simulink model "vis_servo"  (R2020b)
settings: Solver=ode45  StartTime=0.0  StopTime=100  MaxStep=0.5e-3  RelTol=1e-11
InitFcn:
  | init
values from neighbouring files (symbols this model uses):
  C_features_0 = homtrans(inv(W_T_C_0), W_features)    [init.m]
  C_features_desired = inv(O_T_C_desired) * O_features    [init.m]
  Cdesired_T_C0 = inv(C0_T_Cdesired)    [init.m]
  lambdaT_const = 1    [init.m]
  s0 = C_features_0(:)    [init.m]
  Ts = 0.15    [init.m]    (also in test_for_c.m = 0.1)
  vMax = .5    (= 0.5)    [init.m]
  W_p_C_0 = W_T_C_0.transl'    [init.m]
  W_q_C_0 = rotm2quat(W_T_C_0.R)    [init.m]
  wMax = deg2rad(20)    [init.m]
settings Model: Creator=marco  LastModifiedBy=marco

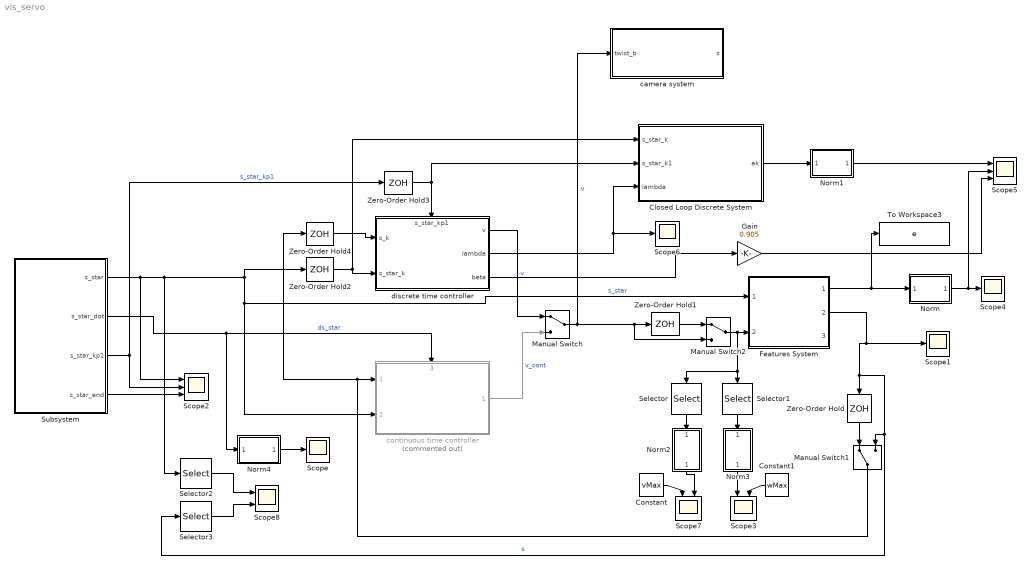
== system vis_servo ==
  Closed Loop Discrete System : Subsystem  mask{forward_action_enabled=on, Ts=Ts, e0=e0*0}
  Constant : Constant  Value=vMax
  Constant1 : Constant  Value=wMax
  Features System : Subsystem  ReferencedSubsystem=Features_System  s0=s0
  Gain : Gain  Gain=0.905
  Manual Switch : ManualSwitch
  Manual Switch1 : ManualSwitch
  Manual Switch2 : ManualSwitch
  Norm{,1..4} (5 alike) : Subsystem  ReferencedSubsystem=Norm
  Scope{,1,4,6} (4 alike) : Scope
  Scope2 : Scope  NumInputPorts=3
  Scope3 : Scope  NumInputPorts=2
  Scope5 : Scope  NumInputPorts=3
  Scope7 : Scope  NumInputPorts=2
  Scope8 : Scope  NumInputPorts=2
  Selector : Selector  InputPortWidth=6  IndexOptions=Index vector (dialog)  Indices=1:3  OutputSizes=1
  Selector1 : Selector  InputPortWidth=6  IndexOptions=Index vector (dialog)  Indices=4:6  OutputSizes=1
  Selector2 : Selector  InputPortWidth=numel(s0)  IndexOptions=Index vector (dialog)  Indices=1:3  OutputSizes=1
  Selector3 : Selector  InputPortWidth=numel(s0)  IndexOptions=Index vector (dialog)  Indices=1:3  OutputSizes=1
  Subsystem : Subsystem  mask{C_features_0=C_features_0, C_features_desired=C_features_desired, Cdesired_T_C0=Cdesired_T_C0.double, Ts=Ts, no_traj=off}
      mask prompts: C_features_0 "C_features_0 (initial features in camera frame)"; C_features_desired "C_features_desired (desired features in camera frame)"; Cdesired_T_C0 "Cdesired_T_C0 (camera initial frame w.r.t. camera desired frame)"
      mask Display:
      | disp('Ref Generator','texmode', 'on')
      | 
      | port_label('output',1,'s^*','texmode', 'on')
      | port_label('output',2,'ds^*','texmode', 'on')
      | port_label('output',3,'s^*_{k+1}','texmode', 'on')
      | port_label('output',4,'s^*_{END}','texmode', 'on')
  To Workspace3 : ToWorkspace  VariableName=e  SaveFormat=Timeseries  SampleTime=0.001
  Zero-Order Hold{,1..4} (5 alike) : ZeroOrderHold  SampleTime=Ts
  camera system : Subsystem
  continuous time controller : Subsystem  Commented=on  ReferencedSubsystem=continuous_time_controller  lambda=lambda_const  forward_action_enabled=off
      settings: PortSchema="{\"entries\":[{\"content\":{\"sides\":[{\"content\":{\"connectorIds\":[\"In1\",\"In2\"]},\"type\":\"ConnectorPlacement.EquallySpacedRectSide\",\"uuid\":\"e89226d4-baa4-4c30-af13-ff098f2ce7fc\"},{\"content\":{\"connectorIds\":[\"Out1\"],\"side\":\"RIGHT\"},\"type\":\"ConnectorPlacement.EquallySpacedRectSide\",\"uuid\":\"9d8bce32-3e74-4b83-8e79-37f4d5184f5a\"},{\"content\":{\"connectorIds\":[\"In3\"],\"side\":\"TOP\"},\"type\":\"ConnectorPlacement.EquallySpacedRectSide\",\"uuid\":\"9322580e-0316-476d-a1f3-db89d995a642\"},{\"content\":{\"connectorIds\":[],\"side\":\"HIDDEN\"},\"type\":\"ConnectorPlacement.EquallySpacedRectSide\",\"uuid\":\"a71e587c-d25e-434f-ae20-c6224730a5c7\"}]},\"type\":\"ConnectorPlacement.EquallySpacedConnector\",\"uuid\":\"c231d1ba-4204-4ba1-a9fd-ba17f6d657c2\"}],\"packageUris\":[\"http://schema.mathworks.com/mf0/Connector/R2020b\"],\"version\":\"1.0\"}"
  discrete time controller : Subsystem  mask{Ts=Ts, forward_action_enabled=on, vMax=vMax + inf, wMax=wMax + inf, use_majorant=off, use_lambda_const=on, lambdaT_const=lambdaT_const/2, use_max_analytic_lambda=off}
      settings: PortSchema="{\"entries\":[{\"content\":{\"sides\":[{\"content\":{\"connectorIds\":[\"In1\",\"In2\"]},\"type\":\"ConnectorPlacement.EquallySpacedRectSide\",\"uuid\":\"e89226d4-baa4-4c30-af13-ff098f2ce7fc\"},{\"content\":{\"connectorIds\":[\"Out1\",\"Out2\",\"Out3\"],\"side\":\"RIGHT\"},\"type\":\"ConnectorPlacement.EquallySpacedRectSide\",\"uuid\":\"9d8bce32-3e74-4b83-8e79-37f4d5184f5a\"},{\"content\":{\"connectorIds\":[\"In3\"],\"side\":\"TOP\"},\"type\":\"ConnectorPlacement.EquallySpacedRectSide\",\"uuid\":\"9322580e-0316-476d-a1f3-db89d995a642\"},{\"content\":{\"connectorIds\":[],\"side\":\"HIDDEN\"},\"type\":\"ConnectorPlacement.EquallySpacedRectSide\",\"uuid\":\"a71e587c-d25e-434f-ae20-c6224730a5c7\"}]},\"type\":\"ConnectorPlacement.EquallySpacedConnector\",\"uuid\":\"c231d1ba-4204-4ba1-a9fd-ba17f6d657c2\"}],\"packageUris\":[\"http://schema.mathworks.com/mf0/Connector/R2020b\"],\"version\":\"1.0\"}"
      mask Display:
      | disp('Discrete Time Controller','texmode', 'on')
      | 
      | port_label('output',1,'v_k','texmode', 'on')
      | port_label('output',2,'\lambda_k','texmode', 'on')
      | port_label('output',3,'\beta_k','texmode', 'on')
      | port_label('input',1,'s_k','texmode', 'on')
      | port_label('input',2,'s^*_k','texmode', 'on')
      | port_label('input',3,'s^*_{k+1}','texmode', 'on')
  wires:
  Features System/2 -> Scope1/1, Selector3/1, Manual Switch1/2, Zero-Order Hold/1  "s"
  Manual Switch/1 -> Manual Switch2/2, Zero-Order Hold1/1, camera system/1(twist_b)  "v"
  discrete time controller/1(v) -> Manual Switch/1  "v"
  continuous time controller/1 -> Manual Switch/2  "v_cont"
  Subsystem/1(s_star) -> Scope2/1, Selector2/1, Zero-Order Hold2/1, continuous time controller/2, Features System/1  "s_star"
  Subsystem/2(s_star_dot) -> Norm4/1, continuous time controller/3  "ds_star"
  Subsystem/3(s_star_kp1) -> Zero-Order Hold3/1, Scope2/2  "s_star_kp1"
  Features System/1 -> To Workspace3/1, Norm/1
  Norm/1 -> Scope5/2, Scope4/1
  Manual Switch1/1 -> Zero-Order Hold4/1, continuous time controller/1
  Zero-Order Hold/1 -> Manual Switch1/1
  Zero-Order Hold1/1 -> Manual Switch2/1
  Manual Switch2/1 -> Selector1/1, Selector/1, Features System/2
  Zero-Order Hold2/1 -> Closed Loop Discrete System/1(s_star_k), discrete time controller/2(s_star_k)
  Zero-Order Hold4/1 -> discrete time controller/1(s_k)
  discrete time controller/2(lambda) -> Closed Loop Discrete System/3(lambda), Scope6/1
  Closed Loop Discrete System/1(ek) -> Norm1/1
  Norm1/1 -> Scope5/1
  Zero-Order Hold3/1 -> discrete time controller/3(s_star_kp1), Closed Loop Discrete System/2(s_star_k1)
  Subsystem/4(s_star_end) -> Scope2/3
  Selector/1 -> Norm2/1
  Selector1/1 -> Norm3/1
  Norm3/1 -> Scope3/1
  Norm2/1 -> Scope7/2
  Constant/1 -> Scope7/1
  Constant1/1 -> Scope3/2
  Selector2/1 -> Scope8/1
  Selector3/1 -> Scope8/2
  discrete time controller/3(beta) -> Gain/1
  Gain/1 -> Scope5/3
  Norm4/1 -> Scope/1

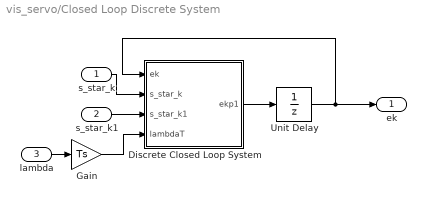
== system vis_servo/Closed Loop Discrete System ==
  s_star_k : Inport
  s_star_k1 : Inport  Port=2
  lambda : Inport  Port=3
  Discrete Closed Loop System : MATLAB Function  TreatAsAtomicUnit=on
  Gain : Gain  Gain=Ts
  Unit Delay : UnitDelay  InitialCondition=e0  SampleTime=Ts  HasFrameUpgradeWarning=on
  ek : Outport
  wires:
  Discrete Closed Loop System/1(ekp1) -> Unit Delay/1
  s_star_k/1 -> Discrete Closed Loop System/2(s_star_k)
  s_star_k1/1 -> Discrete Closed Loop System/3(s_star_k1)
  Gain/1 -> Discrete Closed Loop System/4(lambdaT)
  Unit Delay/1 -> ek/1, Discrete Closed Loop System/1(ek)
  lambda/1 -> Gain/1

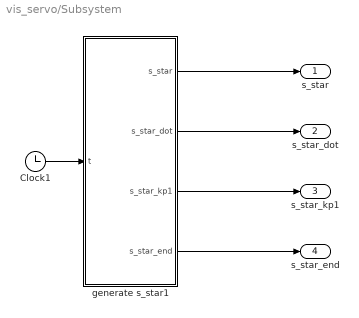
== system vis_servo/Subsystem ==
  Clock1 : Clock
  generate s_star1 : MATLAB Function  TreatAsAtomicUnit=on
  s_star : Outport
  s_star_dot : Outport  Port=2
  s_star_kp1 : Outport  Port=3
  s_star_end : Outport  Port=4
  wires:
  Clock1/1 -> generate s_star1/1(t)
  generate s_star1/3(s_star_kp1) -> s_star_kp1/1
  generate s_star1/1(s_star) -> s_star/1
  generate s_star1/2(s_star_dot) -> s_star_dot/1
  generate s_star1/4(s_star_end) -> s_star_end/1

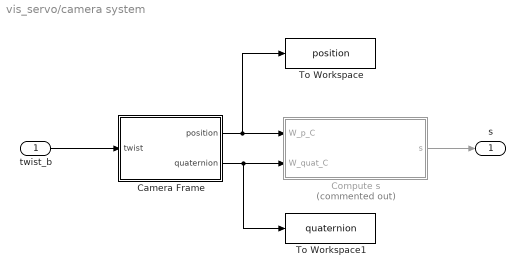
== system vis_servo/camera system ==
  twist_b : Inport
  Camera Frame : Subsystem
  Compute s : MATLAB Function  Commented=on  TreatAsAtomicUnit=on
  To Workspace : ToWorkspace  VariableName=position  SaveFormat=Timeseries  SampleTime=0.001
  To Workspace1 : ToWorkspace  VariableName=quaternion  SaveFormat=Timeseries  SampleTime=0.001
  s : Outport
  wires:
  Compute s/1(s) -> s/1
  twist_b/1 -> Camera Frame/1(twist)
  Camera Frame/2(quaternion) -> Compute s/2(W_quat_C), To Workspace1/1
  Camera Frame/1(position) -> Compute s/1(W_p_C), To Workspace/1

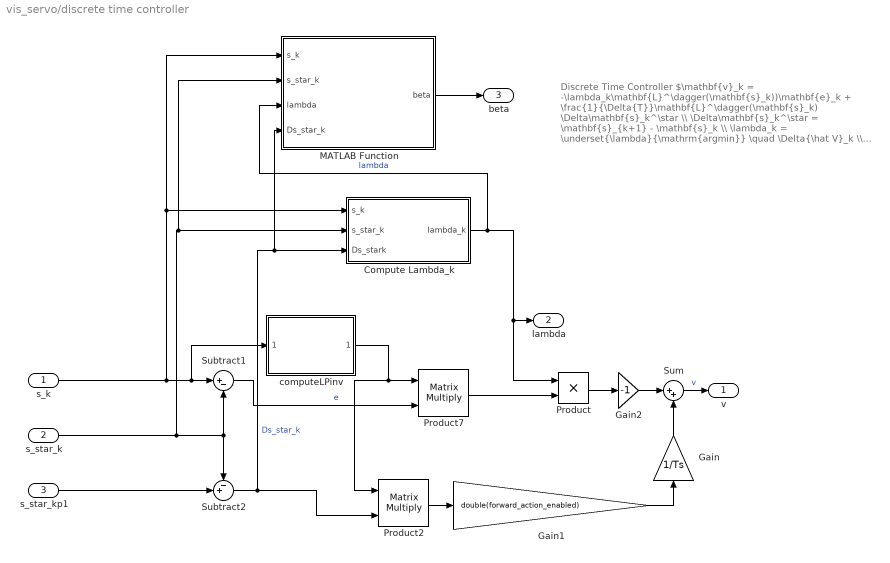
== system vis_servo/discrete time controller ==
  note: Discrete Time Controller
      | $\mathbf{v}_k = -\lambda_k\mathbf{L}^\dagger(\mathbf{s}_k))\mathbf{e}_k + \frac{1}{\Delta{T}}\mathbf{L}^\dagger(\mathbf{s}_k) \Delta\mathbf{s}_k^\star \\ \Delta\mathbf{s}_k^\star = \mathbf{s}_{k+1} - \mathbf{s}_k \\ \lambda_k = \underset{\lambda}{\mathrm{argmin}} \quad \Delta{\hat V}_k \\ \textrm{s.t.} \quad \textrm{velocity limits}$
  s_k : Inport
  s_star_k : Inport  Port=2
  s_star_kp1 : Inport  Port=3
  Compute Lambda_k : Subsystem
  Gain : Gain  Gain=1/Ts
  Gain1 : Gain  Gain=double(forward_action_enabled)
  Gain2 : Gain  Gain=-1
  MATLAB Function : MATLAB Function  TreatAsAtomicUnit=on
  Product : Product
  Product2 : Product  Multiplication=Matrix(*)
  Product7 : Product  Multiplication=Matrix(*)
  Subtract1 : Sum  Inputs=|+-
  Subtract2 : Sum  Inputs=-+|
  Sum : Sum  Inputs=|++
  computeLPinv : Subsystem  ReferencedSubsystem=computeLPinv
  v : Outport
  lambda : Outport  Port=2
  beta : Outport  Port=3
  wires:
  Product2/1 -> Gain1/1
  Subtract2/1 -> MATLAB Function/4(Ds_star_k), Compute Lambda_k/3(Ds_stark), Product2/2  "Ds_star_k"
  Subtract1/1 -> Product7/2  "e"
  s_star_k/1 -> MATLAB Function/2(s_star_k), Compute Lambda_k/2(s_star_k), Subtract2/1, Subtract1/2
  s_k/1 -> MATLAB Function/1(s_k), Compute Lambda_k/1(s_k), computeLPinv/1, Subtract1/1
  Compute Lambda_k/1(lambda_k) -> MATLAB Function/3(lambda), lambda/1, Product/1  "lambda"
  Product/1 -> Gain2/1
  Gain2/1 -> Sum/1
  Product7/1 -> Product/2
  Sum/1 -> v/1  "v"
  s_star_kp1/1 -> Subtract2/2
  Gain/1 -> Sum/2
  Gain1/1 -> Gain/1
  computeLPinv/1 -> Product7/1, Product2/1
  MATLAB Function/1(beta) -> beta/1

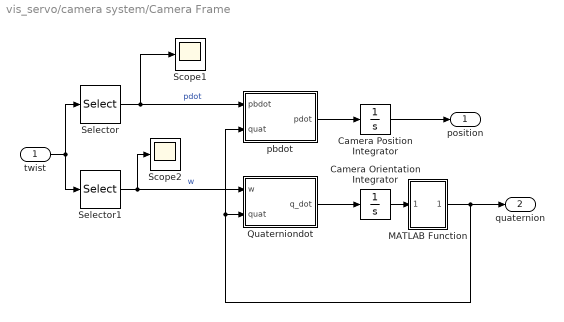
== system vis_servo/camera system/Camera Frame ==
  twist : Inport
  Camera Orientation Integrator : Integrator  InitialCondition=W_q_C_0
  Camera Position Integrator : Integrator  InitialCondition=W_p_C_0
  MATLAB Function : MATLAB Function  TreatAsAtomicUnit=on
  Quaterniondot : MATLAB Function  TreatAsAtomicUnit=on
  Scope1 : Scope
  Scope2 : Scope
  Selector : Selector  InputPortWidth=6  IndexOptions=Index vector (dialog)  Indices=[1:3]  OutputSizes=1
  Selector1 : Selector  InputPortWidth=6  IndexOptions=Index vector (dialog)  Indices=[4:6]  OutputSizes=1
  pbdot : MATLAB Function  TreatAsAtomicUnit=on
  position : Outport
  quaternion : Outport  Port=2
  wires:
  MATLAB Function/1(quat) -> Quaterniondot/2(quat), pbdot/2(quat), quaternion/1
  pbdot/1(pdot) -> Camera Position Integrator/1
  Camera Orientation Integrator/1 -> MATLAB Function/1("quat ")
  Quaterniondot/1(q_dot) -> Camera Orientation Integrator/1
  Camera Position Integrator/1 -> position/1
  Selector1/1 -> Quaterniondot/1(w), Scope2/1  "w"
  Selector/1 -> pbdot/1(pbdot), Scope1/1  "pdot"
  twist/1 -> Selector1/1, Selector/1

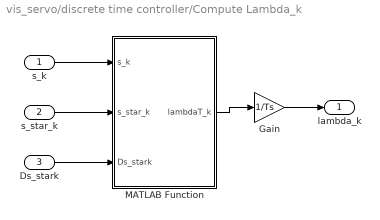
== system vis_servo/discrete time controller/Compute Lambda_k ==
  s_k : Inport
  s_star_k : Inport  Port=2
  Ds_stark : Inport  Port=3
  Gain : Gain  Gain=1/Ts
  MATLAB Function : MATLAB Function  TreatAsAtomicUnit=on
  lambda_k : Outport
  wires:
  s_k/1 -> MATLAB Function/1(s_k)
  s_star_k/1 -> MATLAB Function/2(s_star_k)
  Ds_stark/1 -> MATLAB Function/3(Ds_stark)
  MATLAB Function/1(lambdaT_k) -> Gain/1
  Gain/1 -> lambda_k/1

== matlab function vis_servo/Closed Loop Discrete System/Discrete Closed Loop System ==
  data: ek input; ekp1 output; s_star_k input; s_star_k1 input; lambdaT input; forward_action_enabled parameter boolean
function ekp1 = fcn(ek,s_star_k,s_star_k1,lambdaT,forward_action_enabled)

sk = ek + s_star_k;
Ds_stark = s_star_k1-s_star_k;
L = computeL(sk);
ekp1 = discreteErrorSystemClosedLoop_internal( ...
    lambdaT, ...
    ek, ...
    L, ...
    pinv(L), ...
    Ds_stark, ...
    forward_action_enabled...
    );

== matlab function vis_servo/discrete time controller/MATLAB Function ==
  data: s_k input; beta output; s_star_k input; lambda input; Ds_star_k input; Ts parameter
function beta = computeBeta(s_k,s_star_k, lambda, Ds_star_k, Ts)

e = s_k - s_star_k;

L = computeL(s_k);
Lpinv = pinv(L);
eI = L*Lpinv*e;

if(norm(e) < 10*eps)
    alpha = 1;
else
    alpha = norm(e)/norm(eI);
    if 1-alpha < 1e-5
        alpha = 1;
    end
end
if(alpha < 1)
    dummy = 0;
end

vel1 = - Lpinv*e + Lpinv*Ds_star_k/(lambda*Ts);
% vel1 = - Lpinv*e;
omega1 = vel1(4:6);

a = -2*lambda*Ts*(1-alpha*lambda*Ts*.5*norm(omega1)-.5*lambda*Ts);
b = 2*alpha*(sqrt(alpha^2-1) + lambda*Ts*.5*norm(omega1)*(alpha+lambda*Ts*(1+lambda*Ts*.5*norm(omega1))));
c = alpha^2*Ts*((1+lambda*Ts*.5*norm(omega1))^2);

DELTA = b^2 - 4*a*c;
if(DELTA < 0)
   beta = 0;
   return;
end
sol1 = (-b - sqrt(DELTA))/2*a;
sol2 = (-b + sqrt(DELTA))/2*a;

if sol1*sol2 <= 0
   beta = max(sol1,sol2); 
   return; % OK
end

if sol1 < 0
    beta = 0; % both negative impossible
    return;
end

% if sol1 > 0
   beta = max(sol1,sol2); % impossible
   return;
% end

== matlab function vis_servo/discrete time controller/Compute Lambda_k/MATLAB Function ==
  data: s_k input; lambdaT_k output; s_star_k input; Ds_stark input; Ts parameter double; vMax parameter double; wMax parameter double; forward_action_enabled parameter boolean; use_majorant parameter boolean; use_lambda_const parameter boolean; lambdaT_const parameter double; use_max_analytic_lambda parameter boolean
function lambdaT_k = fcn(s_k, s_star_k, Ds_stark, Ts, vMax, wMax, forward_action_enabled, use_majorant, use_lambda_const, lambdaT_const, use_max_analytic_lambda)
coder.extrinsic('opt_problem_lambdaT'); % <- Informing the Coder

if use_lambda_const
    lambdaT_k = lambdaT_const;
    return;
end

ek = s_k-s_star_k;

if use_max_analytic_lambda
   lambdaT_k = computeAnaliticLambdaTMax(ek,computeL(s_k));
   return;
end


% lambdaT_k = opt_problem_lambdaT(...
%     ek,...
%     s_star_k,...
%     Ts,...
%     vMax,...
%     wMax,...
%     Ds_stark,...
%     forward_action_enabled,...
%     use_majorant...
%     );

lambdaT_k = opt_problem_lambdaT(...
    ek, ...
    s_star_k, ...
    vMax*Ts, ...
    wMax*Ts, ...
    Ds_stark, ...
    forward_action_enabled, ...
    use_majorant ...
    );

== matlab function vis_servo/Subsystem/generate s_star1 ==
  data: t input; s_star output; s_star_dot output; s_star_kp1 output; C_features_0 parameter double; s_star_end output; C_features_desired parameter double; Cdesired_T_C0 parameter double; Ts parameter double; no_traj parameter boolean
function [s_star,s_star_dot, s_star_kp1, s_star_end] = fcn(t, C_features_0, C_features_desired, Cdesired_T_C0, Ts, no_traj)

if no_traj
    s_star = C_features_desired(:);
    s_star_kp1 = C_features_desired(:);
    s_star_dot = zeros(size(s_star));
    s_star_end = C_features_desired(:);
    return
end

% common
pos_ti = 2;
ang_ti = 2;
useQuintic = true;
% trapz
pos_vmax = 0.5;
pos_ai = 0.5;
pos_af = 0.5;
w_max = deg2rad(10);
ang_ai = deg2rad(10);
ang_af = deg2rad(10);
% quintic
pos_tf = pos_ti + (1/pos_vmax);
[~, ~, deltaAng] = quatInterp(t, [1 0 0 0], rotm2quat(Cdesired_T_C0(1:3,1:3)), @(t, deltaAng)trapezVelTraj(t,0,deltaAng,w_max,ang_ai,ang_af,ang_ti));
ang_tf = ang_ti + (deltaAng/w_max);

if useQuintic
    scalarTrajPos = @(t)quinticTraj(t,0,1,pos_ti,pos_tf);
    scalarTrajQuat = @(t,deltaAng)quinticTraj(t,0,deltaAng,ang_ti,ang_tf);
else
    scalarTrajPos = @(t)trapezVelTraj(t,0,1,pos_vmax,pos_ai,pos_af,pos_ti);
    scalarTrajQuat = @(t, deltaAng)trapezVelTraj(t,0,deltaAng,w_max,ang_ai,ang_af,ang_ti);
end

t_kp1 = t + Ts;

initial_quat = [1 0 0 0];
pi = [0;0;0];

final_quat = rotm2quat(Cdesired_T_C0(1:3,1:3));
pf = Cdesired_T_C0(1:3,4);

[Qt, wt] = quatInterp(t, initial_quat, final_quat, scalarTrajQuat);
Rt = quat2rotm(Qt);
[Qt_kp1] = quatInterp(t_kp1, initial_quat, final_quat, scalarTrajQuat);
Rt_kp1 = quat2rotm(Qt_kp1);
% Rt = Cdesired_T_C0(1:3,1:3);
% wt = [0 0 0]';

[pt, ptdot] = positionInterp(t, pi, pf, scalarTrajPos);
[pt_kp1] = positionInterp(t_kp1, pi, pf, scalarTrajPos);
% pt = Cdesired_T_C0(1:3,4);
% ptdot = [0 0 0]';

Tt = [Rt, pt; 0 0 0 1];
Tt_kp1 = [Rt_kp1, pt_kp1; 0 0 0 1];

FEATURE_star = homtrans(Tt, C_features_0);
FEATURE_star_kp1 = homtrans(Tt_kp1, C_features_0);
FEATURE_star_dot = zeros(size(FEATURE_star));
for i=1:size(C_features_0,2)
    FEATURE_star_dot(:,i) = skew(wt)*Rt*C_features_0(:,i) + ptdot(:);
%     FEATURE_star_dot(:,i) = Rt*skew(wt)*FEATURE_star(:,i) + ptdot(:);
end

s_star = FEATURE_star(:);
s_star_kp1 = FEATURE_star_kp1(:);
s_star_dot = FEATURE_star_dot(:);
s_star_end = C_features_desired(:);

== matlab function vis_servo/camera system/Camera Frame/MATLAB Function ==
  data: quat input; quat output
function quat = fcn(quat)

quat = unit(quat);

== matlab function vis_servo/camera system/Camera Frame/Quaterniondot ==
  data: w input; q_dot output; quat input
function q_dot = fcn(w, quat)

q_dot = quat_dotb(quat,w);
% Q = UnitQuaternion(quat);
% Q_dot = Q.dot(w);
% q_dot = Q_dot.double'; 
% q_dot = [0 0 0 0]';

== matlab function vis_servo/camera system/Camera Frame/pbdot ==
  data: pbdot input; pdot output; quat input
function pdot = fcn(pbdot, quat)

W_R_B = quat2rotm(quat');
pdot = W_R_B*pbdot;

== matlab function vis_servo/camera system/Compute s ==
  data: W_p_C input; s output; W_quat_C input; params parameter
function s = fcn(W_p_C, W_quat_C, params)

% W_T_C = SE3(quat2rotm(W_quat_C'),W_p_C);
W_T_C = [quat2rotm(W_quat_C'), W_p_C; 0 0 0 1];

% C_features = inv(W_T_C) * params.W_T_O * params.O_features;
C_features = homtrans(inv(W_T_C) * params.W_T_O, params.O_features);

s = C_features(:);

% s = params.O_features(:);
